simulink model "sim_greenderivative"  (R2019b)
settings: Solver=FixedStepAuto  StartTime=0.0  StopTime=50  FixedStep=0.05  RelTol=1e-3
settings Model: Creator=greg  LastModifiedBy=greg

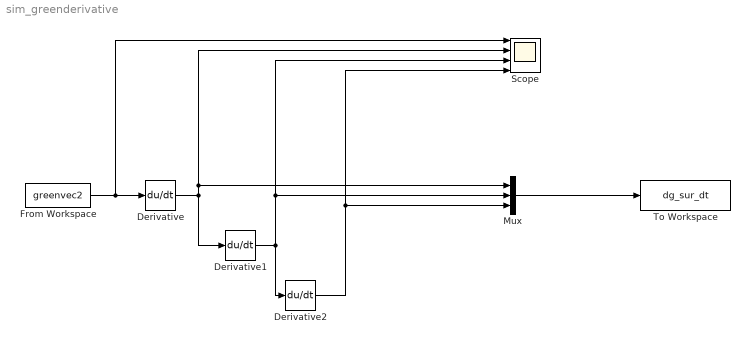
== system sim_greenderivative ==
  Derivative : Derivative
  Derivative1 : Derivative
  Derivative2 : Derivative
  From Workspace : FromWorkspace  VariableName=greenvec2  SampleTime=0.05
  Mux : Mux  Inputs=3
  Scope : Scope  NumInputPorts=4
  To Workspace : ToWorkspace  VariableName=dg_sur_dt  SampleTime=-1
  wires:
  From Workspace/1 -> Scope/1, Derivative/1
  Derivative/1 -> Mux/1, Scope/2, Derivative1/1
  Derivative1/1 -> Mux/2, Scope/3, Derivative2/1
  Derivative2/1 -> Mux/3, Scope/4
  Mux/1 -> To Workspace/1
